simulink model "test"  (Simulink 8.5)
settings: Solver=ode45  StartTime=0.0  StopTime=1000.0  RelTol=1e-3
model workspace: external: MATLAB Code (data not in the file)
undefined symbols (not defined in the file): EbNo
libraries: commdigbbndam3 x2, commchan3 x1, commsink2 x1, commutil2 x1, commrandsrc2 x1
settings Model: Creator=francisco  LastModifiedBy=francisco
settings DataIOCC: SignalLoggingSaveFormat=Dataset
settings OptimizationCC: ExpressionDepthLimit=128
settings DebuggingCC: UnderspecifiedInitializationDetection=Simplified  MergeDetectMultiDrivingBlocksExec=error  FcnCallInpInsideContextMsg=EnableAllAsError  StateNameClashWarn=none
settings GRTTargetCC: CombineOutputUpdateFcns=on  GRTInterface=off

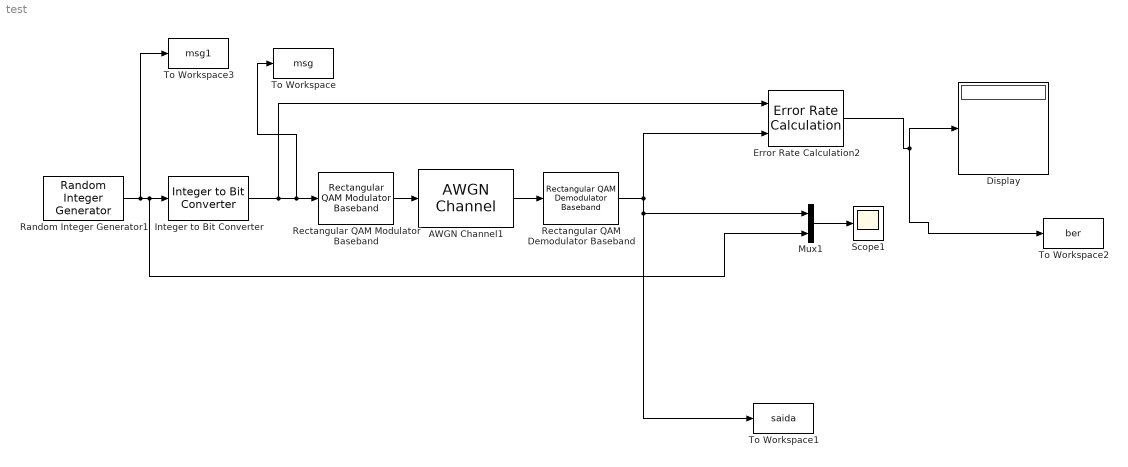
== system test ==
  AWGN Channel1 : commchan3/AWGN Channel  InputProcessing=Columns as channels (frame based)  seed=67  noiseMode="Signal to noise ratio  (Eb/No)"  EbNodB=15  EsNodB=EbNo+10*log10(6)  SNRdB=10  bitsPerSym=2  Ps=1  Tsym=1  variance=1
  Display : Display
  Error Rate Calculation2 : commsink2/Error Rate Calculation  N=0  st_delay=0  cp_mode=Entire frame  subframe=[]  PMode=Port  WsName=ErrorVec  RsMode2=off  stop=off  numErr=100  maxBits=1e6
  Integer to Bit Converter : commutil2/Integer to Bit Converter  nbits=2  signedInputValues=Unsigned  bitOrder=MSB first  outDtype=Inherit via internal rule
  Mux1 : Mux  Inputs=2
  Random Integer Generator1 : commrandsrc2/Random Integer Generator  RequirementInfo="{}  %GIDa_f806ea20_e19a_4035_a8ac_7d6336cc0989"  mul=2  seed=37  Ts=1  frameBased=off  sampPerFrame=1  orient=off  outDataType=double
  Rectangular QAM Demodulator Baseband : commdigbbndam3/Rectangular QAM Demodulator Baseband  M=4  PowType=Average Power  MinDist=2  AvgPow=1  PeakPow=1  Ph=0  Dec=Gray  Mapping=[0:15]  OutType=Bit  DecType=Hard decision  VarSource=Dialog  Variance=1  outDtype1=Inherit via internal rule  outDtype2=Inherit via internal rule  derotateFactorWordLen=16  denormFactorWordLen=16  prodOutWordLen=32  prodOutRoundingMode=Floor  prodOutOverflowMode=Wrap  sumWordLen=32
  Rectangular QAM Modulator Baseband : commdigbbndam3/Rectangular QAM Modulator Baseband  M=4  InType=Bit  Enc=Gray  Mapping=[0:15]  PowType=Average Power  MinDist=2  AvgPow=1  PeakPow=1  Ph=0  outDtype=double  outWordLen=16  outUDDataType=sfix(16)  outFracLenMode=Best precision  outFracLen=15
  Scope1 : Scope
      settings: SaveName=ScopeData2  Decimation=100
  To Workspace : ToWorkspace  VariableName=msg  SaveFormat=Timeseries  SampleTime=-1
  To Workspace1 : ToWorkspace  VariableName=saida  SaveFormat=Timeseries  SampleTime=-1
  To Workspace2 : ToWorkspace  VariableName=ber  SampleTime=-1
      settings: MaxDataPoints=1  Save2DSignal=2-D array (concatenate along first dimension)
  To Workspace3 : ToWorkspace  VariableName=msg1  SaveFormat=Timeseries  SampleTime=-1
  wires:
  Random Integer Generator1/1 -> To Workspace3/1, Mux1/2, Integer to Bit Converter/1
  Mux1/1 -> Scope1/1
  Rectangular QAM Modulator Baseband/1 -> AWGN Channel1/1
  Error Rate Calculation2/1 -> To Workspace2/1, Display/1
  AWGN Channel1/1 -> Rectangular QAM Demodulator Baseband/1
  Integer to Bit Converter/1 -> Error Rate Calculation2/1, Rectangular QAM Modulator Baseband/1, To Workspace/1
  Rectangular QAM Demodulator Baseband/1 -> To Workspace1/1, Mux1/1, Error Rate Calculation2/2
